simulink library "lib_global_brake_ctrl_nodiv"  (Simulink 7.7)
settings: Solver=ode45  SolverMode=SingleTasking  StartTime=0.0  StopTime=10.0  RelTol=1e-3
undefined symbols (not defined in the file): distrib
settings Model: Creator=yt59680  LastModifiedBy=lfeng

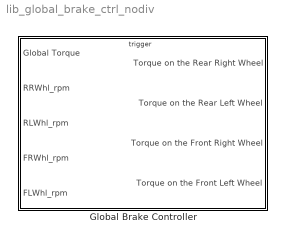
== system lib_global_brake_ctrl_nodiv ==
  Global Brake Controller : Subsystem  TreatAsAtomicUnit=on

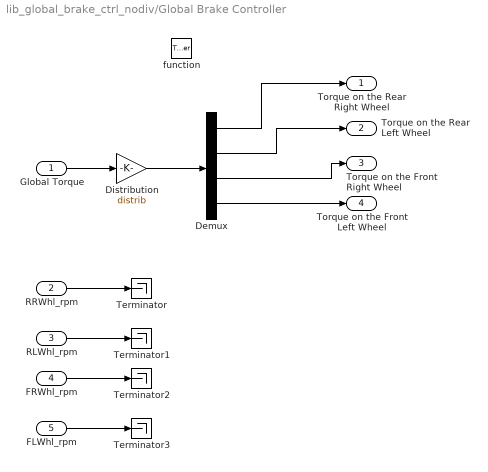
== system lib_global_brake_ctrl_nodiv/Global Brake Controller ==
  Global Torque : Inport
  RRWhl_rpm : Inport  Port=2
  RLWhl_rpm : Inport  Port=3
  FRWhl_rpm : Inport  Port=4
  FLWhl_rpm : Inport  Port=5
  function : TriggerPort  TriggerType=function-call
  Demux : Demux
  Distribution : Gain  Gain=distrib  OutMax=2000  OutDataTypeStr=double
  Terminator{,1..3} (4 alike) : Terminator
  Torque on the Rear Right Wheel : Outport
  Torque on the Rear Left Wheel : Outport  Port=2
  Torque on the Front Right Wheel : Outport  Port=3
  Torque on the Front Left Wheel : Outport  Port=4
  wires:
  FLWhl_rpm/1 -> Terminator3/1
  FRWhl_rpm/1 -> Terminator2/1
  RLWhl_rpm/1 -> Terminator1/1
  RRWhl_rpm/1 -> Terminator/1
  Global Torque/1 -> Distribution/1
  Distribution/1 -> Demux/1
  Demux/4 -> Torque on the Front Left Wheel/1
  Demux/1 -> Torque on the Rear Right Wheel/1
  Demux/2 -> Torque on the Rear Left Wheel/1
  Demux/3 -> Torque on the Front Right Wheel/1
